simulink model "fin_simu_continuous2022a"  (R2022a)
settings: Solver=VariableStepAuto  StartTime=0.0  StopTime=time  RelTol=1e-3
values from neighbouring files (symbols this model uses):
  A = [0.7, 0.2; 0, 0.5]    [code_simu.m]    (also in code_simu_continuous.m)
  A0 = [0, 1; -1, -1.4]    [code_simu_continuous.m]
  B = [1; 0.5]    [code_simu.m]    (also in code_simu_continuous.m)
  B0 = [0; 1]    [code_simu_continuous.m]
  C = [0.2, 0.8]    [code_simu.m]    (also in code_simu_continuous.m)
  C0 = [1, 0]    [code_simu_continuous.m]
  D = [0]    [code_simu.m]    (also in code_simu_continuous.m)
  D0 = [0]    [code_simu_continuous.m]
  omega = 3.14159265*5    (= 15.70796325)    [code_simu.m]    (also in code_simu_continuous.m)
  rho = 0.101    [code_simu.m]    (also in code_simu_continuous.m)
  seed = 17    [code_simu.m]    (also in code_simu_continuous.m)
  sig = 0.001    [code_simu.m]    (also in code_simu_continuous.m)
  ts = 0.005    [code_simu.m]    (also in code_simu_continuous.m)
  wav = 0.7    [code_simu.m]    (also in code_simu_continuous.m)
undefined symbols (not defined in the file or in its folder): AA, b0, b1, b2, b3, BB, CC, DD, w0, w1, w2, w3
settings Model: Creator=IDS_PC  LastModifiedBy=IDS_PC_2023_02

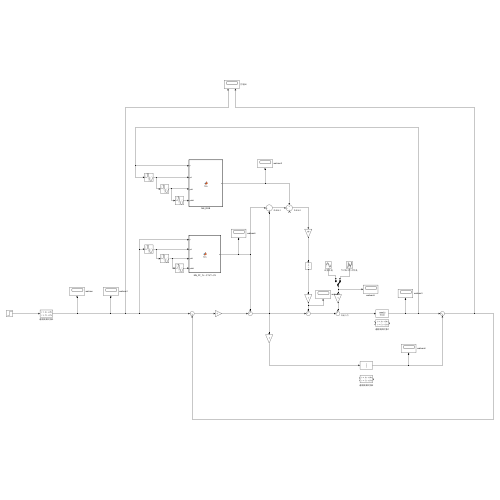
[thumbnail: Simulink's stored preview of the top-level diagram]
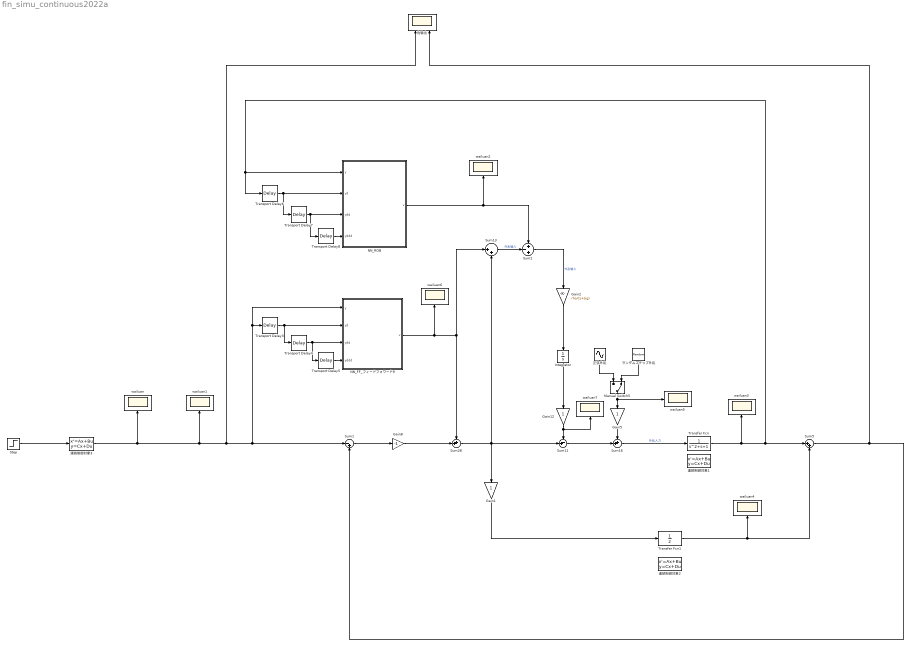
== system fin_simu_continuous2022a ==
  " 正弦外乱" : Sin  Amplitude=wav  Bias=1  Frequency=omega  Phase=1  SampleTime=ts
  Gain1 : Gain
  Gain12 : Gain
  Gain2 : Gain  Gain=rho/(1+sig)
  Gain5 : Gain
  Gain8 : Gain  Gain=-1
  Integrator : Integrator
  Manual Switch5 : ManualSwitch  CurrentSetting=0
  NN_FF_フィードフォワード9 : MATLAB Function  TreatAsAtomicUnit=on
  NN_ROB : MATLAB Function  TreatAsAtomicUnit=on
  Step : Step  SampleTime=0
  Sum1 : Sum  Inputs=|-+
  Sum11 : Sum  Inputs=-+|
  Sum13 : Sum  Inputs=|++
  Sum16 : Sum  Inputs=++|
  Sum2 : Sum  Inputs=+-+
  Sum28 : Sum  Inputs=++|
  Sum5 : Sum  Inputs=|++
  Transfer Fcn : TransferFcn  Denominator=[1 1 1]
  Transfer Fcn1 : TransferFcn  Denominator=[2]
  Transport Delay{3..8} (6 alike) : TransportDelay  DelayTime=ts
  wailuan{,1..7} (8 alike) : Scope
  ランダムステップ外乱 : UniformRandomNumber  Minimum=-wav  Maximum=wav  Seed=seed+5  SampleTime=16
  伪输出 : Scope  NumInputPorts=2
  連続制御対象1 : StateSpace  A=A  B=B  C=C  D=D  InitialCondition=0
  連続制御対象2 : StateSpace  A=AA  B=BB  C=CC  D=DD  InitialCondition=0
  連続制御対象3 : StateSpace  A=A0  B=B0  C=C0  D=D0  InitialCondition=0
  wires:
  Sum16/1 -> Transfer Fcn/1  "外乱入力"
  Gain5/1 -> Sum16/1
  Manual Switch5/1 -> Gain5/1, wailuan5/1
  ランダムステップ外乱/1 -> Manual Switch5/2
  " 正弦外乱"/1 -> Manual Switch5/1
  Sum11/1 -> Sum16/2
  Gain12/1 -> wailuan7/1, Sum11/1
  Sum28/1 -> Sum11/2, Sum13/2, Gain1/1
  Transfer Fcn/1 -> Transport Delay6/1, NN_ROB/1(y), Sum5/1, wailuan3/1
  Gain8/1 -> Sum28/2
  連続制御対象3/1 -> wailuan/1, wailuan1/1, NN_FF_フィードフォワード9/1(y), Transport Delay3/1, Sum1/1, 伪输出/1
  Sum1/1 -> Gain8/1
  Sum5/1 -> 伪输出/2, Sum1/2
  NN_FF_フィードフォワード9/1(v) -> wailuan6/1, Sum13/1, Sum28/1
  NN_ROB/1(v) -> Sum2/1, wailuan2/1
  Sum13/1 -> Sum2/2  "外乱输入"
  Gain2/1 -> Integrator/1
  Sum2/1 -> Gain2/1  "外乱输入"
  Integrator/1 -> Gain12/1
  Transport Delay5/1 -> NN_FF_フィードフォワード9/4(yddd)
  Transport Delay4/1 -> Transport Delay5/1, NN_FF_フィードフォワード9/3(ydd)
  Transport Delay3/1 -> Transport Delay4/1, NN_FF_フィードフォワード9/2(yd)
  Transport Delay8/1 -> NN_ROB/4(yddd)
  Transport Delay6/1 -> Transport Delay7/1, NN_ROB/2(yd)
  Transport Delay7/1 -> Transport Delay8/1, NN_ROB/3(ydd)
  Gain1/1 -> Transfer Fcn1/1
  Transfer Fcn1/1 -> Sum5/2, wailuan4/1
  Step/1 -> 連続制御対象3/1

== matlab function fin_simu_continuous2022a/NN_ROB ==
  data: y input; yd input; ydd input; yddd input; v output; w0 parameter; w1 parameter; w2 parameter; w3 parameter; b0 parameter; b1 parameter; b2 parameter; b3 parameter
function v = fcn(y, yd, ydd, yddd, w0, w1, w2, w3, b0, b1, b2, b3)

    x = [yddd, ydd, yd, y];
    x = x.';

    s1= (transpose(w0)) * x + b0;
    x1= max(0,s1);     %relu 
    s2= (transpose(w1)) * x1 + b1;
    x2= max(0,s2);     %relu
    s3= (transpose(w2)) * x2 + b2;
    x3= max(0,s3);     %relu
    s4= (transpose(w3)) * x3 + b3;

v=s4;

== matlab function fin_simu_continuous2022a/NN_FF_フィードフォワード9 ==
  data: y input; yd input; ydd input; yddd input; v output; w0 parameter; w1 parameter; w2 parameter; w3 parameter; b0 parameter; b1 parameter; b2 parameter; b3 parameter
function v = fcn(y, yd, ydd, yddd, w0, w1, w2, w3, b0, b1, b2, b3)

    x = [yddd, ydd, yd, y];
    x = x.';

    s1= (transpose(w0)) * x + b0;
    x1= max(0,s1);     %relu 
    s2= (transpose(w1)) * x1 + b1;
    x2= max(0,s2);     %relu
    s3= (transpose(w2)) * x2 + b2;
    x3= max(0,s3);     %relu
    s4= (transpose(w3)) * x3 + b3;

v=s4;
